simulink model "test_idealPumpMotor"  (R2013a)
settings: Solver=ode45  StartTime=0.0  StopTime=10.0  RelTol=1e-3
undefined symbols (not defined in the file): rev
libraries: fl_lib x8, nesl_utility x4, usask_hyd_lib x3
settings Model: Creator=tkw954  LastModifiedBy=tkw954
settings SimscapeCC: SimscapeLogType=all  SimscapeLogLimitData=off

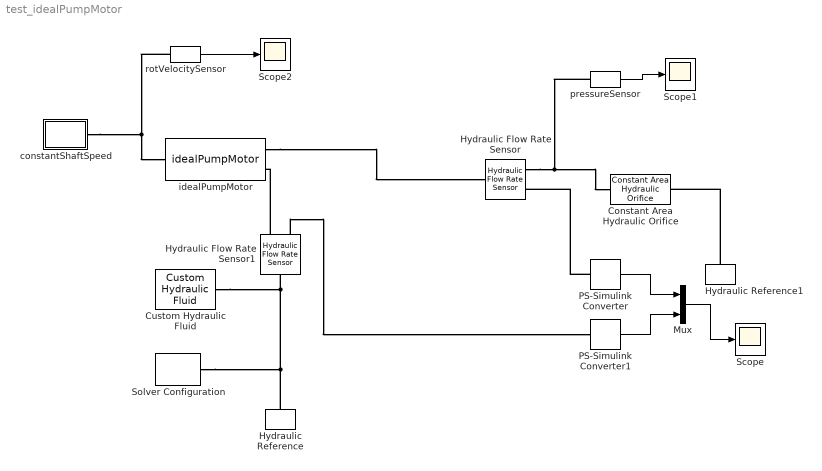
== system test_idealPumpMotor ==
  Constant Area Hydraulic Orifice : fl_lib/Hydraulic/Hydraulic Elements/Constant Area Hydraulic Orifice  area=1e-4 m^2  C_d=0.7  Re_cr=12  C_d_lam=0.0408  D_h=0.0113 m  q_Log=off  p_Log=off  LocalVarNames=|q|p  LocalVarDescs=|q|p  LocalVarLogging=[0 0]
  Custom Hydraulic Fluid : fl_lib/Hydraulic/Hydraulic Utilities/Custom Hydraulic Fluid  density=850 kg/m^3  viscosity_kin=18e-6 m^2/s  bulk=0.8e9 Pa  alpha=0.005  LocalVarLogging=[]
  Hydraulic Flow Rate Sensor : fl_lib/Hydraulic/Hydraulic Sensors/Hydraulic Flow Rate Sensor  q_Log=off  p_Log=off  LocalVarNames=|q|p  LocalVarDescs=|q|p  LocalVarLogging=[0 0]
  Hydraulic Flow Rate Sensor1 : fl_lib/Hydraulic/Hydraulic Sensors/Hydraulic Flow Rate Sensor  q_Log=off  p_Log=off  LocalVarNames=|q|p  LocalVarDescs=|q|p  LocalVarLogging=[0 0]
  Hydraulic Reference : fl_lib/Hydraulic/Hydraulic Elements/Hydraulic Reference  q_Log=off  LocalVarNames=|q  LocalVarDescs=|q  LocalVarLogging=0
  Hydraulic Reference1 : fl_lib/Hydraulic/Hydraulic Elements/Hydraulic Reference  q_Log=off  LocalVarNames=|q  LocalVarDescs=|q  LocalVarLogging=0
  Mux : Mux  Inputs=2
  PS-Simulink Converter : nesl_utility/PS-Simulink Converter  PhysicalDomain=network_engine_domain  SubClassName=ps_output  LeftPortType=input  RightPortType=output  PseudoPeriodic=off  Frequencies=[]  Unit=1  AffineConversion=off
  PS-Simulink Converter1 : nesl_utility/PS-Simulink Converter  PhysicalDomain=network_engine_domain  SubClassName=ps_output  LeftPortType=input  RightPortType=output  PseudoPeriodic=off  Frequencies=[]  Unit=1  AffineConversion=off
  Scope : Scope
  Scope1 : Scope
  Scope2 : Scope
      settings: SaveName=ScopeData2
  Solver Configuration : nesl_utility/Solver Configuration  PhysicalDomain=network_engine_domain  SubClassName=solver  LeftPortType=input  RightPortType=generic  Accelerate=off  Tones=[]  Harmonics=[]  SimulateNoise=off  Profile=off  UseLocalSampling=off  EnableSwitchedLinearOptims=on  FrequencyDomain=off  UseCCode=off  UseNewInitialization=off  DoDC=off  ResidualTolerance=1e-09  UseLocalSolver=off  LocalSolverChoice=NE_BACKWARD_EULER_ADVANCER  LocalSolverSampleTime=0.001  DoFixedCost=off  MaxNonlinIter=3  MaxModeIter=2  LinearAlgebra=Sparse  DelaysMemoryBudget=1024
  constantShaftSpeed : Subsystem  mask(Constant Shaft Speed){w_rpm=1750}
      mask prompts: w_rpm "Shaft speed (rev/min)"
      mask help: Outputs constant shaft speed.
      mask Display:
      | color('red')
      | port_label('rconn',1,'S')
  idealPumpMotor : usask_hyd_lib/idealPumpMotor  D=200e-6
  pressureSensor : usask_hyd_lib/pressureSensor  unitNum=kPa
  rotVelocitySensor : usask_hyd_lib/rotVelocitySensor  unitNum=rev/min
  wires:
  PS-Simulink Converter/1 -> Mux/1
  PS-Simulink Converter1/1 -> Mux/2
  Mux/1 -> Scope/1
  pressureSensor/1 -> Scope1/1
  rotVelocitySensor/1 -> Scope2/1
  connections:
  Hydraulic Reference/LConn1 -- Solver Configuration/RConn1 -- Custom Hydraulic Fluid/RConn1 -- Hydraulic Flow Rate Sensor1/LConn1
  Hydraulic Reference1/LConn1 -- Constant Area Hydraulic Orifice/RConn1
  Hydraulic Flow Rate Sensor/RConn2 -- pressureSensor/LConn1 -- Constant Area Hydraulic Orifice/LConn1
  PS-Simulink Converter/LConn1 -- Hydraulic Flow Rate Sensor/RConn1
  Hydraulic Flow Rate Sensor1/RConn2 -- idealPumpMotor/RConn1
  Hydraulic Flow Rate Sensor1/RConn1 -- PS-Simulink Converter1/LConn1
  idealPumpMotor/RConn2 -- Hydraulic Flow Rate Sensor/LConn1
  rotVelocitySensor/LConn1 -- idealPumpMotor/LConn1 -- constantShaftSpeed/RConn1

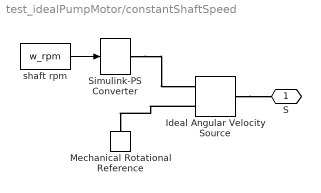
== system test_idealPumpMotor/constantShaftSpeed ==
  Ideal Angular Velocity Source : fl_lib/Mechanical/Mechanical Sources/Ideal Angular Velocity Source  w_Log=off  t_Log=off  LocalVarNames=|w|t  LocalVarDescs=|w|t  LocalVarLogging=[0 0]
  Mechanical Rotational Reference : fl_lib/Mechanical/Rotational Elements/Mechanical Rotational Reference  t_Log=off  LocalVarNames=|t  LocalVarDescs=|t  LocalVarLogging=0
  Simulink-PS Converter : nesl_utility/Simulink-PS Converter  PhysicalDomain=network_engine_domain  SubClassName=ps_input  LeftPortType=input  RightPortType=output  PseudoPeriodic=off  Frequencies=[]  NoiseDistribution=none  NoiseParameters=[]  Unit=rpm  AffineConversion=off  InputFiltering=off  SimscapeFilterOrder=1  InputFilterTimeConstant=0.001  UdotUserProvided=1
  shaft rpm : Constant  Value=w_rpm
  S : PMIOPort  Port=1  Side=Right
  wires:
  shaft rpm/1 -> Simulink-PS Converter/1
  connections:
  Ideal Angular Velocity Source/LConn1 -- S/RConn1
  Ideal Angular Velocity Source/RConn2 -- Mechanical Rotational Reference/LConn1
  Simulink-PS Converter/RConn1 -- Ideal Angular Velocity Source/RConn1
